simulink model "ConvertisseurSigmaDelta"  (R2017a)
settings: Solver=ode3  StartTime=0.0  StopTime=Tsim  FixedStep=TsR  RelTol=1e-3  EnableMultiTasking=on
values from neighbouring files (symbols this model uses):
  gk = ones(1,L)/(L)    [mConvertisseurSigmaDelta.m]
  nu0 = 10    [mConvertisseurSigmaDelta.m]    (also in mModulateurSigmaDelta.m)
  Tsn = 1/nusn    (= 0.001)    [mConvertisseurSigmaDelta.m]    (also in mModulateurSigmaDelta.m = 0.002)
undefined symbols (not defined in the file or in its folder): A, B
settings Model: ExtModeTrigMode=oneshot  ExtModeArmWhenConnect=off  Creator=gscorlet  LastModifiedBy=telep
settings DataIOCC: SaveFormat=Array  SignalLoggingSaveFormat=ModelDataLogs
settings OptimizationCC: BlockReduction=off  BooleanDataType=off  ExpressionDepthLimit=2147483647  LifeSpan=inf
settings DebuggingCC: SaveWithParameterizedLinksMsg=none  UnderspecifiedInitializationDetection=Classic  MergeDetectMultiDrivingBlocksExec=none  SignalResolutionControl=TryResolveAllWithWarning  MultiTaskDSMMsg=warning  MultiTaskCondExecSysMsg=none  FcnCallInpInsideContextMsg=warning  StateNameClashWarn=warning  SFUnexpectedBacktrackingDiag=warning  SFNoUnconditionalDefaultTransitionDiag=warning  SFExecutionAtInitializationDiag=none
settings HardwareCC: ProdBitPerPointer=32  ProdBitPerSizeT=32  ProdBitPerPtrDiffT=32  ProdLargestAtomicFloat=None  ProdIntDivRoundTo=Undefined  ProdEndianess=Unspecified  ProdWordSize=32  ProdHWDeviceType=32-bit Generic  TargetUnknown=on
settings ModelReferenceCC: PropagateSignalLabelsOutOfModel=off
settings GRTTargetCC: TargetLangStandard=C89/C90 (ANSI)  GeneratePreprocessorConditionals=Disable all  CombineOutputUpdateFcns=off  GRTInterface=on
settings ConfigComp: CovMetricSettings=dw  CovHtmlReporting=on  CovSaveCumulativeToWorkspaceVar=on  CovSaveSingleToWorkspaceVar=on  CovExternalEMLEnable=off

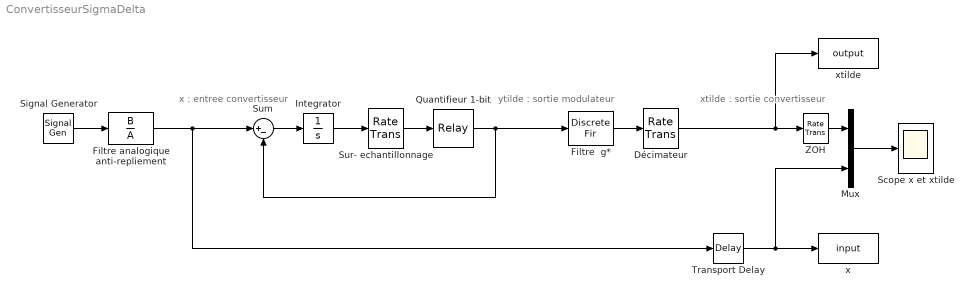
== system ConvertisseurSigmaDelta ==
  note: x : entree
      | convertisseur
  note: ytilde : sortie
      | modulateur
  note: xtilde : sortie
      | convertisseur
  Décimateur : RateTransition  OutPortSampleTime=Tsn
  Filtre  g* : DiscreteFir  Coefficients=gk
  Filtre analogique anti-repliement : TransferFcn  Numerator=B  Denominator=A
  Integrator : Integrator
  Mux : Mux  Inputs=2
  Quantifieur 1-bit : Relay  OffSwitchValue=-eps  OffOutputValue=-1
  Scope x et xtilde : Scope
  Signal Generator : SignalGenerator  WaveForm=sawtooth  Frequency=nu0  VectorParams1D=off
  Sum : Sum  Inputs=|+-  SaturateOnIntegerOverflow=on  InputSameDT=on  OutDataTypeStr=Inherit: Same as first input
  Sur- echantillonnage : RateTransition  OutPortSampleTime=TsR
  Transport Delay : TransportDelay  DelayTime=2*Tsn
  ZOH : RateTransition  OutPortSampleTime=TsR
  x : ToWorkspace  VariableName=input  SaveFormat=Timeseries  SampleTime=-1
  xtilde : ToWorkspace  VariableName=output  SaveFormat=Timeseries  SampleTime=-1
  wires:
  Integrator/1 -> Sur- echantillonnage/1
  Sum/1 -> Integrator/1
  Signal Generator/1 -> Filtre analogique anti-repliement/1
  Mux/1 -> Scope x et xtilde/1
  Sur- echantillonnage/1 -> Quantifieur 1-bit/1
  Quantifieur 1-bit/1 -> Sum/2, Filtre  g*/1
  Filtre  g*/1 -> Décimateur/1
  Décimateur/1 -> ZOH/1, xtilde/1
  Transport Delay/1 -> x/1, Mux/2
  ZOH/1 -> Mux/1
  Filtre analogique anti-repliement/1 -> Sum/1, Transport Delay/1
